simulink model "sampleModel1765"  (R2023a)
settings: Solver=VariableStepAuto  StartTime=0.0  StopTime=10.0  RelTol=1e-3
libraries: hdlsllib x5
settings Model: Creator=user1  LastModifiedBy=user1

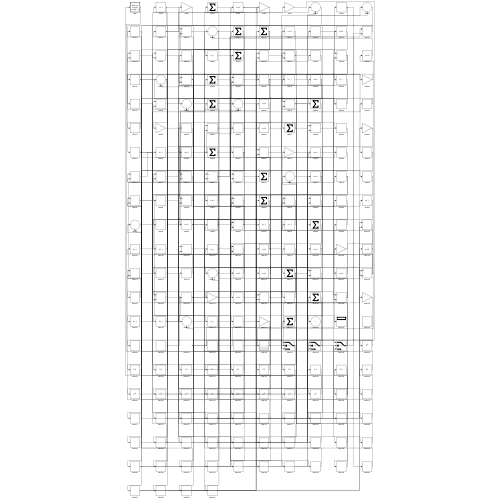
[thumbnail: Simulink's stored preview of the top-level diagram]
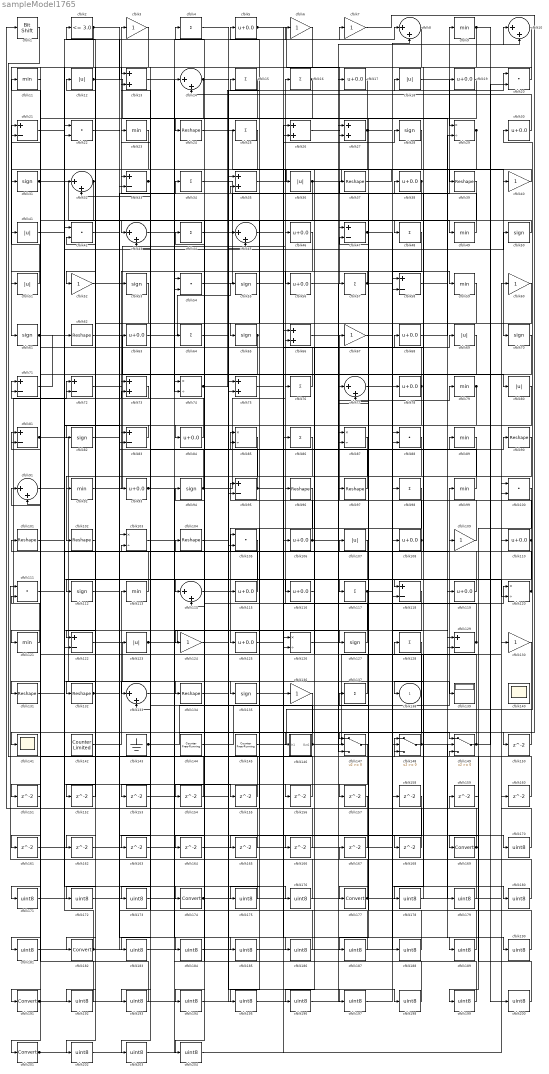
== system sampleModel1765 ==
  cfblk1 : hdlsllib/Logic and Bit Operations/Bit Shift  mode=Shift Left Logical  N=0
  cfblk{8,10,14,32,43,45,77,91,114,133} (10 alike) : Sum  Inputs=|++
  cfblk{20,22,42,54,88,100,105,111} (8 alike) : DotProduct  OutDataTypeStr=Inherit: Inherit via internal rule
  cfblk{24,37,39,62,90,96..97,101..102,104,131..132,134} (13 alike) : Reshape
  cfblk{29,74,85,87,103,120,126} (7 alike) : Product  Inputs=*/  RndMeth=Zero  SaturateOnIntegerOverflow=on
  cfblk{5,17,19,30,38,46,56,63,68,78,84,93,106,108,110,115..116,119,125} (19 alike) : Bias  Bias=0.0  SaturateOnIntegerOverflow=off
  cfblk{12,18,36,41,51,69,80,107,123} (9 alike) : Abs  SaturateOnIntegerOverflow=off
  cfblk{3,6..7,40,52,60,67,109,124,130,136} (11 alike) : Gain
  cfblk{9,11,23,49,59,79,89,92,99,113,121} (11 alike) : MinMax
  cfblk{28,31,50,53,55,61,65,70,82,94,112,127,135} (13 alike) : Signum
  cfblk{4,15..16,25,34,44,48,57,64,76,86,98,117,128,137} (15 alike) : Sum  Inputs=+
  cfblk{21,33,47,58,71..72,81,83,95,118,122,129} (12 alike) : Sum  Inputs=+-
  cfblk{13,26..27,35,66,73,75} (7 alike) : Sum
  cfblk139 : Display
  cfblk140 : Scope
      settings: Floating=on
  cfblk141 : Scope
  cfblk142 : hdlsllib/Sources/Counter Limited  uplimit=7  tsamp=-1
  cfblk143 : Ground
  cfblk144 : hdlsllib/Sources/Counter Free-Running  NumBits=16  tsamp=-1
  cfblk145 : hdlsllib/Sources/Counter Free-Running  NumBits=16  tsamp=-1
  cfblk146 : Subsystem
      settings: LibrarySourceBlock=|
      | hdlsllib/Ports &
      | Subsystems/Subsystem
  cfblk147 : Switch  SaturateOnIntegerOverflow=off  InputSameDT=off
  cfblk148 : Switch  SaturateOnIntegerOverflow=off  InputSameDT=off
  cfblk149 : Switch  SaturateOnIntegerOverflow=off  InputSameDT=off
  cfblk{150..168} (19 alike) : Delay  SampleTime=1
  cfblk{169,174,177,182,191,201} (6 alike) : DataTypeConversion  SaturateOnIntegerOverflow=off  RndMeth=Floor
  cfblk{170..173,175..176,178..181,183..190,192..200,202..204} (30 alike) : DataTypeConversion  OutDataTypeStr=uint8  SaturateOnIntegerOverflow=off  RndMeth=Floor
  cfblk2 : hdlsllib/Logic and Bit Operations/Compare To Constant  relop=<=  const=3.0  OutDataTypeStr=boolean
  cfblk138 : Outport  VectorParamsAs1DForOutWhenUnconnected=off
  wires:
  cfblk117/1 -> cfblk129/2, cfblk165/1, cfblk166/1
  cfblk110/1 -> cfblk67/1, cfblk147/2
  cfblk81/1 -> cfblk134/1, cfblk126/2
  cfblk6/1 -> cfblk61/1
  cfblk144/1 -> cfblk99/1
  cfblk121/1 -> cfblk72/1
  cfblk74/1 -> cfblk18/1, cfblk19/1
  cfblk88/1 -> cfblk182/1
  cfblk71/1 -> cfblk62/1
  cfblk96/1 -> cfblk125/1
  cfblk135/1 -> cfblk120/1
  cfblk31/1 -> cfblk48/1, cfblk135/1
  cfblk109/1 -> cfblk38/1
  cfblk127/1 -> cfblk71/1
  cfblk37/1 -> cfblk70/1
  cfblk104/1 -> cfblk35/1
  cfblk50/1 -> cfblk43/1
  cfblk13/1 -> cfblk74/2
  cfblk14/1 -> cfblk132/1, cfblk147/3
  cfblk108/1 -> cfblk85/2, cfblk204/1
  cfblk97/1 -> cfblk87/1
  cfblk92/1 -> cfblk16/1
  cfblk49/1 -> cfblk3/1
  cfblk17/1 -> cfblk43/2
  cfblk83/1 -> cfblk82/1
  cfblk35/1 -> cfblk40/1
  cfblk94/1 -> cfblk46/1, cfblk13/2
  cfblk111/1 -> cfblk174/1
  cfblk99/1 -> cfblk33/1
  cfblk129/1 -> cfblk76/1, cfblk37/1
  cfblk69/1 -> cfblk121/1
  cfblk54/1 -> cfblk9/1
  cfblk102/1 -> cfblk12/1
  cfblk125/1 -> cfblk28/1
  cfblk145/1 -> cfblk30/1
  cfblk142/1 -> cfblk113/1
  cfblk70/1 -> cfblk131/1
  cfblk124/1 -> cfblk89/1
  cfblk131/1 -> cfblk107/1
  cfblk100/1 -> cfblk169/1
  cfblk5/1 -> cfblk57/1, cfblk118/2
  cfblk24/1 -> cfblk36/1
  cfblk123/1 -> cfblk127/1, cfblk85/1
  cfblk65/1 -> cfblk114/1, cfblk181/1
  cfblk86/1 -> cfblk102/1
  cfblk46/1 -> cfblk93/1
  cfblk42/1 -> cfblk47/1
  cfblk79/1 -> cfblk124/1, cfblk153/1
  cfblk1/1 -> cfblk148/1
  cfblk38/1 -> cfblk187/1, cfblk196/1
  cfblk90/1 -> cfblk92/1
  cfblk78/1 -> cfblk15/1, cfblk146/1(In1), cfblk122/2
  cfblk47/1 -> cfblk108/1, cfblk59/1
  cfblk101/1 -> cfblk50/1
  cfblk9/1 -> cfblk52/1, cfblk200/1
  cfblk53/1 -> cfblk83/1
  cfblk120/1 -> cfblk68/1, cfblk47/2
  cfblk48/1 -> cfblk75/2
  cfblk4/1 -> cfblk45/1
  cfblk72/1 -> cfblk14/1
  cfblk146/1(Out1) -> cfblk110/1, cfblk32/2
  cfblk51/1 -> cfblk21/1
  cfblk33/1 -> cfblk73/1, cfblk63/1
  cfblk20/1 -> cfblk13/1
  cfblk28/1 -> cfblk33/2
  cfblk122/1 -> cfblk139/1
  cfblk62/1 -> cfblk80/1
  cfblk15/1 -> cfblk133/1
  cfblk64/1 -> cfblk115/1
  cfblk29/1 -> cfblk41/1, cfblk156/1
  cfblk73/1 -> cfblk72/2
  cfblk26/1 -> cfblk27/2
  cfblk63/1 -> cfblk55/1
  cfblk75/1 -> cfblk149/1
  cfblk93/1 -> cfblk64/1, cfblk120/2
  cfblk149/1 -> cfblk81/1, cfblk95/1, cfblk20/2
  cfblk132/1 -> cfblk105/1, cfblk34/1
  cfblk91/1 -> cfblk7/1
  cfblk2/1 -> cfblk141/1, cfblk176/1
  cfblk113/1 -> cfblk101/1
  cfblk126/1 -> cfblk109/1
  cfblk136/1 -> cfblk201/1
  cfblk40/1 -> cfblk31/1
  cfblk133/1 -> cfblk8/1
  cfblk36/1 -> cfblk39/1, cfblk65/1, cfblk151/1
  cfblk45/1 -> cfblk66/1
  cfblk12/1 -> cfblk6/1, cfblk119/1
  cfblk34/1 -> cfblk129/1
  cfblk115/1 -> cfblk2/1
  cfblk27/1 -> cfblk91/2, cfblk10/2, cfblk24/1
  cfblk30/1 -> cfblk14/2
  cfblk61/1 -> cfblk83/2, cfblk116/1
  cfblk84/1 -> cfblk73/2
  cfblk10/1 -> cfblk138/1
  cfblk128/1 -> cfblk177/1
  cfblk116/1 -> cfblk66/2
  cfblk18/1 -> cfblk29/1
  cfblk137/1 -> cfblk96/1
  cfblk66/1 -> cfblk10/1
  cfblk57/1 -> cfblk56/1, cfblk20/1
  cfblk32/1 -> cfblk161/1, cfblk162/1
  cfblk112/1 -> cfblk90/1
  cfblk3/1 -> cfblk22/2
  cfblk43/1 -> cfblk49/1
  cfblk143/1 -> cfblk147/1, cfblk86/1
  cfblk95/1 -> cfblk69/1, cfblk4/1
  cfblk23/1 -> cfblk112/1
  cfblk119/1 -> cfblk23/1
  cfblk39/1 -> cfblk84/1
  cfblk106/1 -> cfblk79/1, cfblk5/1
  cfblk16/1 -> cfblk122/1, cfblk51/1
  cfblk76/1 -> cfblk21/2
  cfblk68/1 -> cfblk29/2
  cfblk148/1 -> cfblk123/1, cfblk190/1
  cfblk114/1 -> cfblk117/1
  cfblk56/1 -> cfblk118/1
  cfblk11/1 -> cfblk191/1
  cfblk21/1 -> cfblk32/1
  cfblk7/1 -> cfblk150/1
  cfblk150/1 -> cfblk148/2
  cfblk89/1 -> cfblk152/1
  cfblk152/1 -> cfblk42/2
  cfblk153/1 -> cfblk105/2
  cfblk118/1 -> cfblk154/1
  cfblk154/1 -> cfblk81/2
  cfblk41/1 -> cfblk155/1
  cfblk155/1 -> cfblk74/1
  cfblk156/1 -> cfblk133/2
  cfblk19/1 -> cfblk157/1
  cfblk157/1 -> cfblk1/1
  cfblk160/1 -> cfblk148/3
  cfblk161/1 -> cfblk26/2
  cfblk107/1 -> cfblk163/1
  cfblk163/1 -> cfblk8/2
  cfblk147/1 -> cfblk164/1
  cfblk164/1 -> cfblk27/1
  cfblk165/1 -> cfblk75/1
  cfblk166/1 -> cfblk71/2
  cfblk167/1 -> cfblk22/1
  cfblk82/1 -> cfblk168/1
  cfblk168/1 -> cfblk35/2
  cfblk169/1 -> cfblk149/3, cfblk94/1
  cfblk22/1 -> cfblk170/1
  cfblk170/1 -> cfblk100/1
  cfblk151/1 -> cfblk171/1
  cfblk171/1 -> cfblk100/2
  cfblk60/1 -> cfblk172/1
  cfblk172/1 -> cfblk158/1
  cfblk87/1 -> cfblk173/1
  cfblk173/1 -> cfblk60/1
  cfblk174/1 -> cfblk95/2, cfblk149/2, cfblk104/1
  cfblk158/1 -> cfblk175/1
  cfblk175/1 -> cfblk111/1
  cfblk176/1 -> cfblk111/2
  cfblk177/1 -> cfblk167/1, cfblk137/1
  cfblk59/1 -> cfblk178/1
  cfblk178/1 -> cfblk128/1
  cfblk58/1 -> cfblk179/1
  cfblk179/1 -> cfblk114/2
  cfblk67/1 -> cfblk180/1
  cfblk180/1 -> cfblk58/1
  cfblk181/1 -> cfblk58/2
  cfblk182/1 -> cfblk53/1, cfblk42/1
  cfblk8/1 -> cfblk183/1
  cfblk183/1 -> cfblk88/1
  cfblk162/1 -> cfblk184/1
  cfblk184/1 -> cfblk88/2
  cfblk103/1 -> cfblk185/1
  cfblk185/1 -> cfblk87/2
  cfblk52/1 -> cfblk186/1
  cfblk186/1 -> cfblk103/1
  cfblk187/1 -> cfblk103/2
  cfblk77/1 -> cfblk188/1
  cfblk188/1 -> cfblk97/1
  cfblk55/1 -> cfblk189/1
  cfblk189/1 -> cfblk77/1
  cfblk190/1 -> cfblk77/2
  cfblk191/1 -> cfblk17/1, cfblk45/2
  cfblk80/1 -> cfblk192/1
  cfblk192/1 -> cfblk11/1
  cfblk25/1 -> cfblk193/1
  cfblk193/1 -> cfblk91/1
  cfblk85/1 -> cfblk194/1
  cfblk194/1 -> cfblk25/1
  cfblk98/1 -> cfblk195/1
  cfblk195/1 -> cfblk26/1
  cfblk196/1 -> cfblk98/1
  cfblk44/1 -> cfblk197/1
  cfblk197/1 -> cfblk78/1
  cfblk134/1 -> cfblk198/1
  cfblk198/1 -> cfblk44/1
  cfblk159/1 -> cfblk199/1
  cfblk199/1 -> cfblk54/1
  cfblk200/1 -> cfblk159/1
  cfblk201/1 -> cfblk160/1, cfblk54/2, cfblk106/1
  cfblk105/1 -> cfblk202/1
  cfblk202/1 -> cfblk136/1
  cfblk130/1 -> cfblk203/1
  cfblk203/1 -> cfblk126/1
  cfblk204/1 -> cfblk130/1

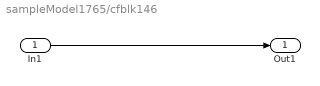
== system sampleModel1765/cfblk146 ==
  In1 : Inport
  Out1 : Outport
  wires:
  In1/1 -> Out1/1
